simulink model "G_System"  (R2018b)
settings: Solver=FixedStepDiscrete  StartTime=0.0  StopTime=10.0  RelTol=1e-3
libraries: simulink x1
settings Model: Creator=Mostafa  LastModifiedBy=Mostafa
settings ConfigSet: Description=Mostafa Hany Imam
settings OptimizationCC: DefaultParameterBehavior=Inlined  EnhancedBackFolding=on  PassReuseOutputArgsAs=Individual arguments  OptimizeBlockOrder=speed  DifferentSizesBufferReuse=on  OptimizationCustomize=off
settings DebuggingCC: UnderspecifiedInitializationDetection=Classic  MergeDetectMultiDrivingBlocksExec=none  ParameterTunabilityLossMsg=error
settings ModelReferenceCC: PropagateSignalLabelsOutOfModel=off
settings SFSimCC: MATLABDynamicMemAlloc=off
settings RTWCC: SystemTargetFile=ert.tlc  GenCodeOnly=on  TemplateMakefile=ert_default_tmf  GenerateReport=on  IncludeHyperlinkInReport=on  LaunchReport=on  GenerateTraceInfo=on  GenerateTraceReport=on  GenerateTraceReportSl=on  GenerateTraceReportSf=on  GenerateTraceReportEml=on
settings CodeAppCC: ForceParamTrailComments=on  IgnoreCustomStorageClasses=off  OperatorAnnotations=on  SimulinkDataObjDesc=on  SFDataObjDesc=on  InsertBlockDesc=on
settings ERTTargetCC: TargetLangStandard=C99 (ISO)  GenerateSampleERTMain=on  InlinedParameterPlacement=NonHierarchical  ERTCustomFileTemplate=example_file_process.tlc

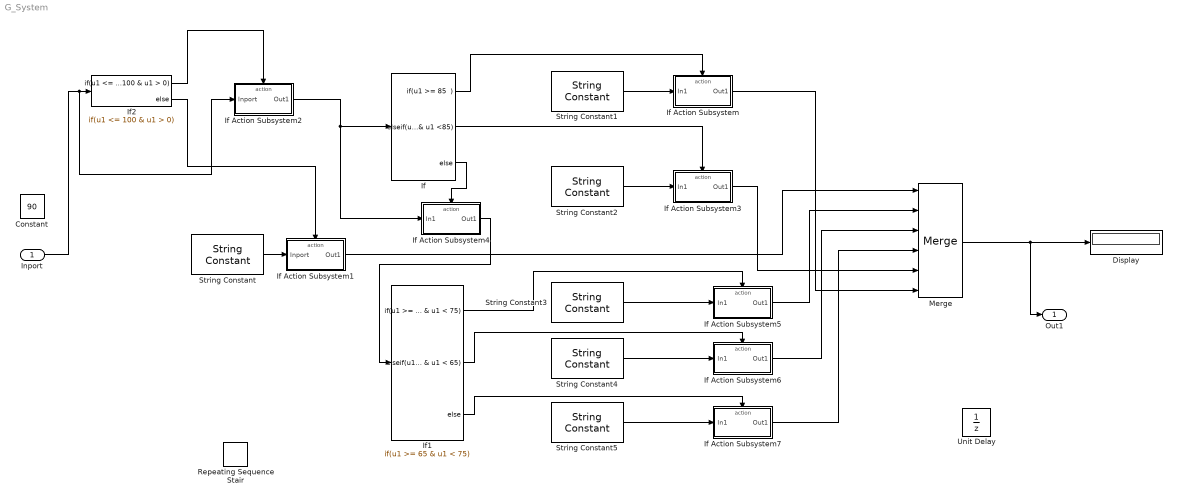
== system G_System ==
  Inport : Inport
  Constant : Constant  Value=90  OutDataTypeStr=uint32
  Display : Display
  If : If  IfExpression=u1 >= 85  ElseIfExpressions=u1 >= 75 & u1 <85
  If Action Subsystem : Subsystem  TreatAsAtomicUnit=on
  If Action Subsystem1 : Subsystem  TreatAsAtomicUnit=on
  If Action Subsystem2 : Subsystem  TreatAsAtomicUnit=on
  If Action Subsystem3 : Subsystem  TreatAsAtomicUnit=on
  If Action Subsystem4 : Subsystem  TreatAsAtomicUnit=on
  If Action Subsystem5 : Subsystem  TreatAsAtomicUnit=on
  If Action Subsystem6 : Subsystem  TreatAsAtomicUnit=on
  If Action Subsystem7 : Subsystem  TreatAsAtomicUnit=on
  If1 : If  IfExpression=u1 >= 65 & u1 < 75  ElseIfExpressions=u1 >=50 & u1 < 65
  If2 : If  IfExpression=u1 <= 100 & u1 > 0
  Merge : Merge  Inputs=6
  "Repeating Sequence Stair " : simulink/Sources/Repeating Sequence Stair  OutValues=[3 1 4 2 1].'  tsamp=-1  OutMin=[]  OutMax=[]  OutDataTypeStr=double  OutputDataTypeScalingMode=double  OutDataType=fixdt(0,8)  ConRadixGroup=Best Precision: Vector-wise  OutScaling=2^-12
  String Constant : StringConstant  String="\"Out of Range\""
  String Constant1 : StringConstant  String="\"Excellent\""
  String Constant2 : StringConstant  String="\"Very Good\""
  String Constant3 : StringConstant  String="\"Good\""
  String Constant4 : StringConstant  String="\"Pass\""
  String Constant5 : StringConstant  String="\"Fail\""
  Unit Delay : UnitDelay  SampleTime=-1
  Out1 : Outport
  wires:
  If2/2 -> If Action Subsystem1/Action
  If2/1 -> If Action Subsystem2/Action
  String Constant/1 -> If Action Subsystem1/1(Inport)
  If Action Subsystem2/1(Out1) -> If Action Subsystem4/1(In1), If/1
  If/1 -> If Action Subsystem/Action
  String Constant1/1 -> If Action Subsystem/1(In1)
  String Constant2/1 -> If Action Subsystem3/1(In1)
  If/2 -> If Action Subsystem3/Action
  If/3 -> If Action Subsystem4/Action
  If Action Subsystem4/1(Out1) -> If1/1
  If1/1 -> If Action Subsystem5/Action
  String Constant3/1 -> If Action Subsystem5/1(In1)
  If1/2 -> If Action Subsystem6/Action
  String Constant4/1 -> If Action Subsystem6/1(In1)
  String Constant5/1 -> If Action Subsystem7/1(In1)
  If1/3 -> If Action Subsystem7/Action
  If Action Subsystem1/1(Out1) -> Merge/1
  If Action Subsystem5/1(Out1) -> Merge/2
  If Action Subsystem6/1(Out1) -> Merge/3
  If Action Subsystem7/1(Out1) -> Merge/4
  If Action Subsystem3/1(Out1) -> Merge/5
  If Action Subsystem/1(Out1) -> Merge/6
  Merge/1 -> Out1/1, Display/1
  Inport/1 -> If Action Subsystem2/1(Inport), If2/1

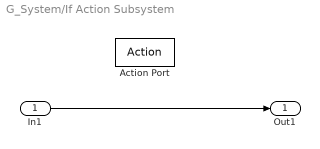
== system G_System/If Action Subsystem ==
  In1 : Inport
  Action Port : ActionPort  ActionType=then
  Out1 : Outport
  wires:
  In1/1 -> Out1/1

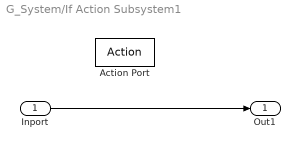
== system G_System/If Action Subsystem1 ==
  Inport : Inport
  Action Port : ActionPort  ActionType=else
  Out1 : Outport
  wires:
  Inport/1 -> Out1/1

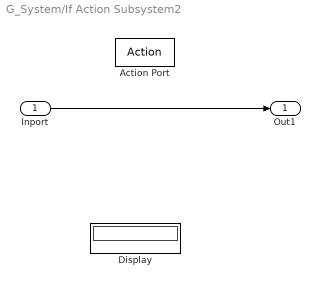
== system G_System/If Action Subsystem2 ==
  Inport : Inport
  Action Port : ActionPort  ActionType=then
  Display : Display
  Out1 : Outport  OutDataTypeStr=uint32
  wires:
  Inport/1 -> Out1/1

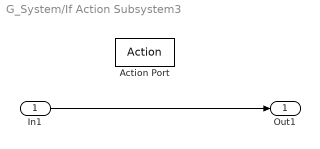
== system G_System/If Action Subsystem3 ==
  In1 : Inport
  Action Port : ActionPort  ActionType=elseif
  Out1 : Outport
  wires:
  In1/1 -> Out1/1

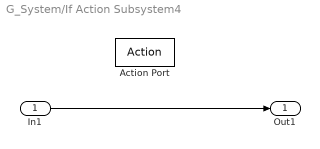
== system G_System/If Action Subsystem4 ==
  In1 : Inport  OutDataTypeStr=uint32
  Action Port : ActionPort  ActionType=else
  Out1 : Outport
  wires:
  In1/1 -> Out1/1

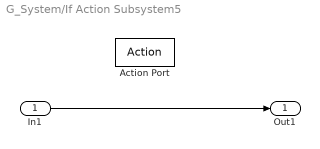
== system G_System/If Action Subsystem5 ==
  In1 : Inport
  Action Port : ActionPort  ActionType=then
  Out1 : Outport
  wires:
  In1/1 -> Out1/1

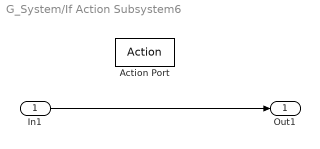
== system G_System/If Action Subsystem6 ==
  In1 : Inport
  Action Port : ActionPort  ActionType=elseif
  Out1 : Outport
  wires:
  In1/1 -> Out1/1

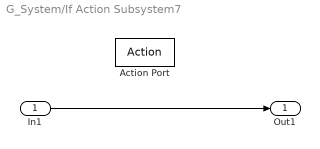
== system G_System/If Action Subsystem7 ==
  In1 : Inport
  Action Port : ActionPort  ActionType=else
  Out1 : Outport
  wires:
  In1/1 -> Out1/1
